simulink model "dblcart1"  (Simulink 6.0)
settings: Solver=ode23  SolverMode=SingleTasking  StartTime=0  StopTime=10000  MaxStep=0.1  RelTol=1e-3  AbsTol=1e-6
PreLoadFcn:
  | load dblcart1
undefined symbols (not defined in the file or in its folder): ae, be, ce, de, ka, m1, m2
settings Model: Creator=The MathWorks Inc.  LastModifiedBy=batserve  ExtModeAutoUpdateStatusClock=off
settings DataIOCC: ExternalInput=[]  InitialState=[]  LimitDataPoints=off  SaveOutput=off  SaveTime=off
settings OptimizationCC: BooleanDataType=off
settings DebuggingCC: CheckExecutionContextPreStartOutputMsg=on  CheckExecutionContextRuntimeOutputMsg=on  SolverPrmCheckMsg=none
settings HardwareCC: TargetUnknown=on

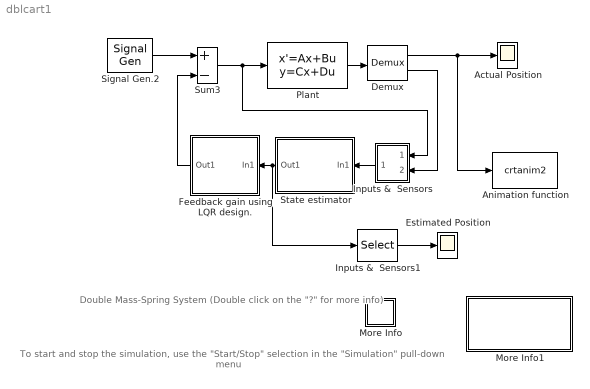
== system dblcart1 ==
  note: Double Mass-Spring System
      | (Double click on the "?" for more info)
  note: To start and stop the simulation, use the "Start/Stop"
      | selection in the "Simulation" pull-down menu
  Actual Position : Scope
      settings: TickLabels=on  TimeRange=40.000000  DataFormat=Array
  Animation function : S-Function  FunctionName=crtanim2  Parameters=0.1
      settings: DeleteFcn=if ~isempty(findobj('type','figure','name','dblcart1 Animation'));close('dblcart1 Animation'); end;
  Demux : Demux  Outputs=[2,1]
  Estimated Position : Scope
      settings: TickLabels=on  TimeRange=40.000000  DataFormat=Array
  Feedback gain using LQR design. : Subsystem  Orientation=left  PropExecContextAcrossSSBoundary=on  mask(Regulator){@1=K}
      mask prompts: @1 "K"
      mask help: Matrix Gain
      mask init:
      | k=@1;
      mask Help: Matrix Gain block
      mask Display: disp('K')
  Inputs &  Sensors : Subsystem  Orientation=left  PropExecContextAcrossSSBoundary=on
  Inputs &  Sensors1 : Selector  Elements=[1 3]  InputPortWidth=4
  More Info : Subsystem  PropExecContextAcrossSSBoundary=on
      mask Display: disp('?')
  More Info1 : Subsystem  PropExecContextAcrossSSBoundary=on
      settings: OpenFcn=simcad(bdroot)
      mask Display: disp('Double click\nhere for\nSIMULINK Help')
  Plant : StateSpace  A=[0 1 0 0; -ka/m1 0 ka/m1 0; 0 0 0 1;ka/m2 0 -ka/m2 0]  B=[0; 1; 0; 0]  C=[1 0 0 0;0 0 1 0;0 0 1 0]  D=zeros(3,1)
  Signal Gen.2 : SignalGenerator  WaveForm=square  Amplitude=15  Frequency=0.300000  Units=rad/sec
  State estimator : Subsystem  Orientation=left  PropExecContextAcrossSSBoundary=on
  Sum3 : Sum  Inputs=+-  SaturateOnIntegerOverflow=on  InputSameDT=on
  wires:
  State estimator/1(Out1) -> Inputs &  Sensors1/1, Feedback gain using LQR design./1(In1)
  Inputs &  Sensors/1(Out1) -> State estimator/1(In1)
  Sum3/1 -> Inputs &  Sensors/1(In1), Plant/1
  Demux/1 -> Actual Position/1, Animation function/1
  Feedback gain using LQR design./1(Out1) -> Sum3/2
  Demux/2 -> Inputs &  Sensors/2(In2)
  Plant/1 -> Demux/1
  Signal Gen.2/1 -> Sum3/1
  Inputs &  Sensors1/1 -> Estimated Position/1

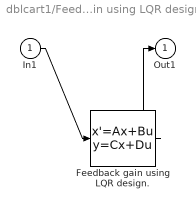
== system dblcart1/Feedback gain using LQR design. ==
  In1 : Inport  Port=1  LatchInput=off
  Feedback gain using LQR design. : StateSpace  A=[]  B=[]  C=[]  D=k
  Out1 : Outport  InitialOutput=0
  wires:
  In1/1 -> Feedback gain using LQR design./1
  Feedback gain using LQR design./1 -> Out1/1

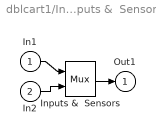
== system dblcart1/Inputs &  Sensors ==
  In1 : Inport  Port=1  LatchInput=off
  In2 : Inport  Port=2  LatchInput=off
  Inputs &  Sensors : Mux  Inputs=2
  Out1 : Outport  InitialOutput=0
  wires:
  In1/1 -> Inputs &  Sensors/1
  In2/1 -> Inputs &  Sensors/2
  Inputs &  Sensors/1 -> Out1/1

== system dblcart1/More Info ==
  note: In this system, the only sensor is attached to the mass
      | on the left, and the actuator is attached to the mass on
      | the left. State estimation and LQR control are used.
  note: Associated with the demo is an animation function that
      | will automatically open a figure window and display to it.
  note: This system models a double spring-mass-damper
      | system with a periodically varying forcing function.

== system dblcart1/More Info1 ==
  note: Try experimenting with different initial conditions for
      | alpha and gamma to see the unusal coupling effects.
  note: Associated with the demo is an animation function that
      | will automatically open a figure window and display to it.
  note: This system models a double pendulum system where
      | the rest state has both pendulums hanging vertically.

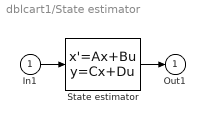
== system dblcart1/State estimator ==
  In1 : Inport  Port=1  LatchInput=off
  State estimator : StateSpace  A=ae  B=be  C=ce  D=de
  Out1 : Outport  InitialOutput=0
  wires:
  In1/1 -> State estimator/1
  State estimator/1 -> Out1/1
